simulink model "qa2b"  (R2018a)
settings: Solver=VariableStepAuto  StartTime=0.0  StopTime=10.0  RelTol=1e-3
libraries: vrlib x2
settings Model: Creator=henry  LastModifiedBy=henry

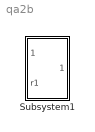
== system qa2b ==
  Subsystem1 : Subsystem  mask(Quaternion Transformation){}
      mask help: This blocks transforms the vector r1 from frame a to frame b.

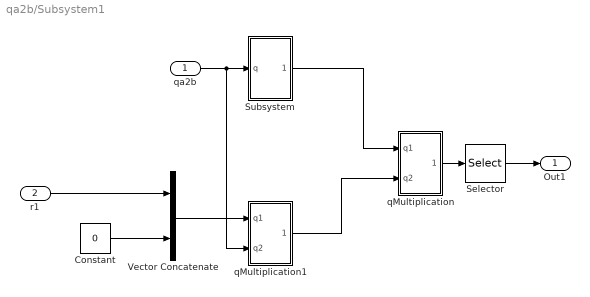
== system qa2b/Subsystem1 ==
  qa2b : Inport
  r1 : Inport  Port=2
  Constant : Constant  Value=0
  Selector : Selector  InputPortWidth=4  IndexOptions=Index vector (dialog)  Indices=[1:3]  OutputSizes=1
  Subsystem : Subsystem  mask(Quaternion Conjugate){}
      mask help: This block takes the conjugate of the input quaternion
  Vector Concatenate : Concatenate
  qMultiplication : Subsystem  mask(Quaternion Multiplication){}
      mask help: This block performs the quaternion multiplication given two input quaternions.
  qMultiplication1 : Subsystem  mask(Quaternion Multiplication){}
      mask help: This block performs the quaternion multiplication given two input quaternions.
  Out1 : Outport
  wires:
  r1/1 -> Vector Concatenate/1
  qa2b/1 -> qMultiplication1/2(q2), Subsystem/1(q)
  Subsystem/1(qConj) -> qMultiplication/1(q1)
  Constant/1 -> Vector Concatenate/2
  Vector Concatenate/1 -> qMultiplication1/1(q1)
  qMultiplication1/1(q12) -> qMultiplication/2(q2)
  qMultiplication/1(q12) -> Selector/1
  Selector/1 -> Out1/1

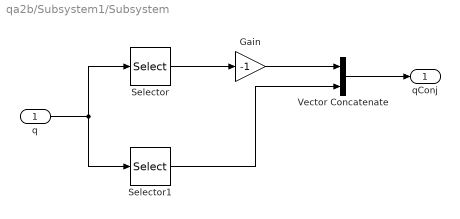
== system qa2b/Subsystem1/Subsystem ==
  q : Inport
  Gain : Gain  Gain=-1
  Selector : Selector  InputPortWidth=4  IndexOptions=Index vector (dialog)  Indices=[1:3]  OutputSizes=1
  Selector1 : Selector  InputPortWidth=4  IndexOptions=Index vector (dialog)  Indices=4  OutputSizes=1
  Vector Concatenate : Concatenate
  qConj : Outport
  wires:
  Selector/1 -> Gain/1
  q/1 -> Selector/1, Selector1/1
  Selector1/1 -> Vector Concatenate/2
  Gain/1 -> Vector Concatenate/1
  Vector Concatenate/1 -> qConj/1

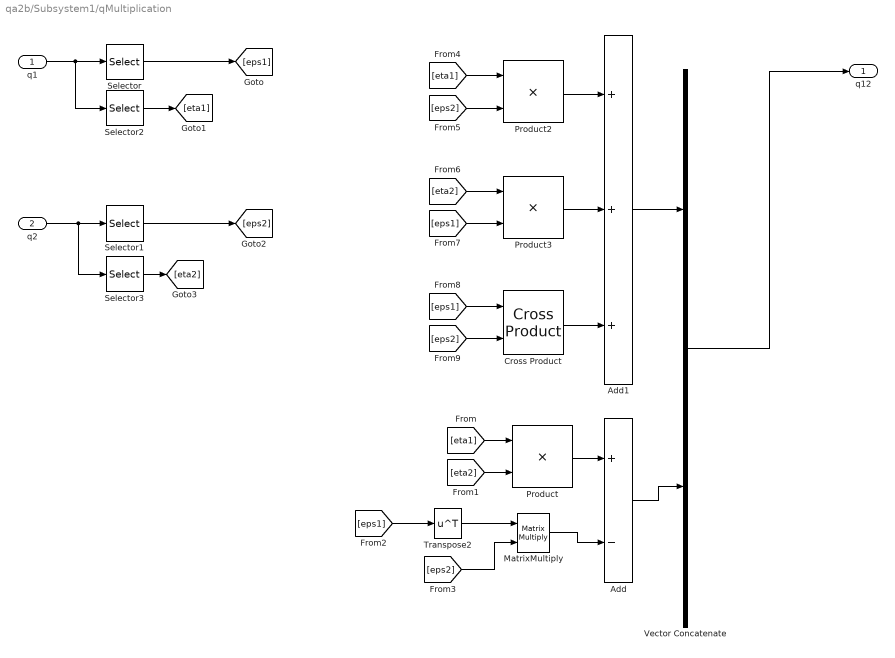
== system qa2b/Subsystem1/qMultiplication ==
  q1 : Inport
  q2 : Inport  Port=2
  Add : Sum  Inputs=+-
  Add1 : Sum  Inputs=+++
  Cross Product : vrlib/Utilities/Cross Product
      settings: SourceProductBaseCode=VR
  MatrixMultiply : Product  Multiplication=Matrix(*)
  Product : Product
  Product2 : Product
  Product3 : Product
  Selector : Selector  InputPortWidth=4  IndexOptions=Index vector (dialog)  Indices=[1:3]  OutputSizes=1
  Selector1 : Selector  InputPortWidth=4  IndexOptions=Index vector (dialog)  Indices=[1:3]  OutputSizes=1
  Selector2 : Selector  InputPortWidth=4  IndexOptions=Index vector (dialog)  Indices=4  OutputSizes=1
  Selector3 : Selector  InputPortWidth=4  IndexOptions=Index vector (dialog)  Indices=4  OutputSizes=1
  Transpose2 : Math  Operator=transpose  SaturateOnIntegerOverflow=on
  Vector Concatenate : Concatenate
  q12 : Outport
  wires:
  Add/1 -> Vector Concatenate/2
  Add1/1 -> Vector Concatenate/1
  [eps2] -> MatrixMultiply/2
  [eps1] -> Cross Product/1
  MatrixMultiply/1 -> Add/2
  [eps2] -> Cross Product/2
  Selector/1 -> [eps1]
  [eps1] -> Product3/2
  [eps2] -> Product2/2
  Vector Concatenate/1 -> q12/1
  [eta1] -> Product/1
  [eta2] -> Product3/1
  q2/1 -> Selector1/1, Selector3/1
  [eps1] -> Transpose2/1
  Cross Product/1 -> Add1/3
  Selector1/1 -> [eps2]
  Selector2/1 -> [eta1]
  Transpose2/1 -> MatrixMultiply/1
  q1/1 -> Selector/1, Selector2/1
  Product3/1 -> Add1/2
  [eta2] -> Product/2
  [eta1] -> Product2/1
  Product/1 -> Add/1
  Product2/1 -> Add1/1
  Selector3/1 -> [eta2]

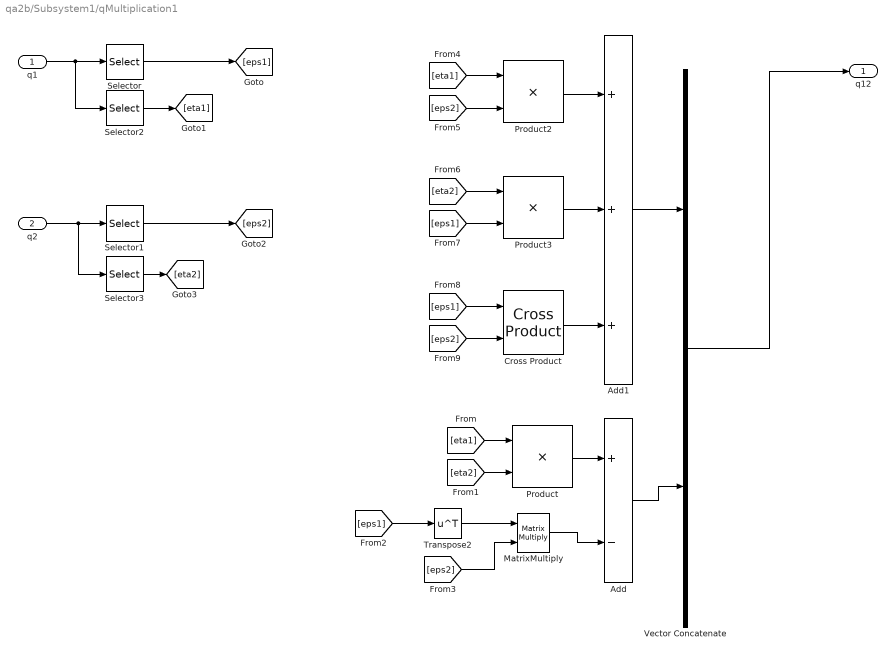
== system qa2b/Subsystem1/qMultiplication1 ==
  q1 : Inport
  q2 : Inport  Port=2
  Add : Sum  Inputs=+-
  Add1 : Sum  Inputs=+++
  Cross Product : vrlib/Utilities/Cross Product
      settings: SourceProductBaseCode=VR
  MatrixMultiply : Product  Multiplication=Matrix(*)
  Product : Product
  Product2 : Product
  Product3 : Product
  Selector : Selector  InputPortWidth=4  IndexOptions=Index vector (dialog)  Indices=[1:3]  OutputSizes=1
  Selector1 : Selector  InputPortWidth=4  IndexOptions=Index vector (dialog)  Indices=[1:3]  OutputSizes=1
  Selector2 : Selector  InputPortWidth=4  IndexOptions=Index vector (dialog)  Indices=4  OutputSizes=1
  Selector3 : Selector  InputPortWidth=4  IndexOptions=Index vector (dialog)  Indices=4  OutputSizes=1
  Transpose2 : Math  Operator=transpose  SaturateOnIntegerOverflow=on
  Vector Concatenate : Concatenate
  q12 : Outport
  wires:
  Selector3/1 -> [eta2]
  Product2/1 -> Add1/1
  Product/1 -> Add/1
  [eta1] -> Product2/1
  [eta2] -> Product/2
  Product3/1 -> Add1/2
  q1/1 -> Selector2/1, Selector/1
  Transpose2/1 -> MatrixMultiply/1
  Selector2/1 -> [eta1]
  Selector1/1 -> [eps2]
  Cross Product/1 -> Add1/3
  [eps1] -> Transpose2/1
  q2/1 -> Selector3/1, Selector1/1
  [eta2] -> Product3/1
  [eta1] -> Product/1
  Vector Concatenate/1 -> q12/1
  [eps2] -> Product2/2
  [eps1] -> Product3/2
  Selector/1 -> [eps1]
  [eps2] -> Cross Product/2
  MatrixMultiply/1 -> Add/2
  [eps1] -> Cross Product/1
  [eps2] -> MatrixMultiply/2
  Add1/1 -> Vector Concatenate/1
  Add/1 -> Vector Concatenate/2
